simulink model "Control_lab2_ex3"  (R2014b)
settings: Solver=ode45  StartTime=0.0  StopTime=10.0  MaxStep=1e-6  RelTol=1e-6
values from neighbouring files (symbols this model uses):
  I = m*(l/2)^2    (= 0.28)    [Control_lab2_ex1.m]    (also in Control_lab2_ex10.m = 0.2; Control_lab2_ex10_2.m = 0.2; Control_lab2_ex2.m = 0.2; Control_lab2_ex3b.m = 0.2)
  Kp = 1    [Control_lab2_ex10.m]    (also in Control_lab2_ex10_2.m; Control_lab2_ex2.m = 140; Control_lab2_ex3b.m = 100; Control_lab2_ex4.m = 100)
  wn = sqrt(m*g*l/(2*I))    [Control_lab2_ex1.m]    (also in Control_lab2_ex10.m; Control_lab2_ex10_2.m; Control_lab2_ex2.m; Control_lab2_ex3b.m)
  xi = c/(2*I*wn)    [Control_lab2_ex1.m]    (also in Control_lab2_ex10.m; Control_lab2_ex10_2.m; Control_lab2_ex2.m; Control_lab2_ex3b.m)
settings Model: Creator=Fei  LastModifiedBy=Fei

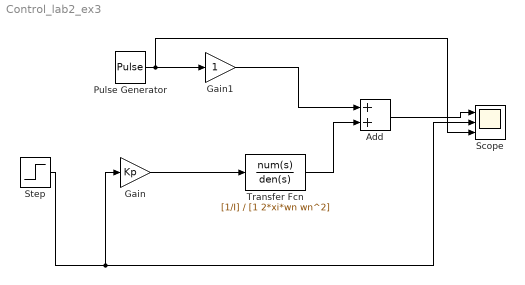
== system Control_lab2_ex3 ==
  Add : Sum
  Gain : Gain  Gain=Kp
  Gain1 : Gain
  Pulse Generator : DiscretePulseGenerator  PulseType=Time based  Amplitude=0.1  Period=1  PulseWidth=50
  Scope : Scope  NumInputPorts=3
      settings: TickLabels=on  YMin=0~-0~0  YMax=16~2~1
  Step : Step  Time=0  SampleTime=0
  Transfer Fcn : TransferFcn  Numerator=[1/I]  Denominator=[1 2*xi*wn wn^2]
  wires:
  Gain/1 -> Transfer Fcn/1
  Step/1 -> Gain/1, Scope/2
  Pulse Generator/1 -> Scope/3, Gain1/1
  Gain1/1 -> Add/1
  Transfer Fcn/1 -> Add/2
  Add/1 -> Scope/1
